simulink model "odev"  (R2020a)
settings: Solver=VariableStepAuto  StartTime=0.0  StopTime=10.0  MaxStep=0.001  RelTol=1e-3
settings Model: Creator=muham  LastModifiedBy=muham

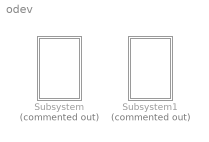
== system odev ==
  Subsystem : Subsystem  Commented=on
  Subsystem1 : Subsystem  Commented=on

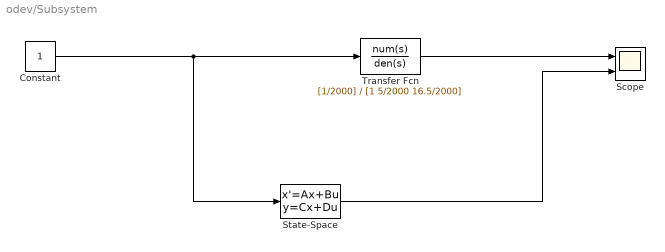
== system odev/Subsystem ==
  Constant : Constant
  Scope : Scope  NumInputPorts=2
  State-Space : StateSpace  A=[0 1; -0.2/12.5,-0.0035/12.5]  B=[0;1/12.5]  C=[1 0]  D=0  InitialCondition=0
  Transfer Fcn : TransferFcn  Numerator=[1/2000]  Denominator=[1 5/2000 16.5/2000]
  wires:
  State-Space/1 -> Scope/2
  Transfer Fcn/1 -> Scope/1
  Constant/1 -> State-Space/1, Transfer Fcn/1

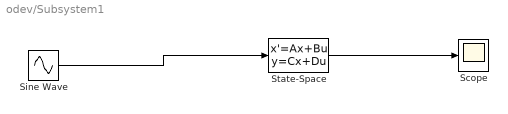
== system odev/Subsystem1 ==
  Scope : Scope
  Sine Wave : Sin  SampleTime=0
  State-Space : StateSpace  A=[0 1 0;0 0 1; -26 -24 -9]  B=[0;0;24]  C=[1 0 0]  D=0  InitialCondition=0
  wires:
  Sine Wave/1 -> State-Space/1
  State-Space/1 -> Scope/1
